simulink model "armonicosv2"  (R2017b)
settings: Solver=VariableStepAuto  StartTime=0.0  StopTime=tsim  MaxStep=stepsize  RelTol=1e-3
values from neighbouring files (symbols this model uses):
  A = blkdiag(matriz{:})    [main.m]
  C = zeros(1,n_arm*2)    [main.m]
  Fs = 500    [main.m]
  HarmonicF1 = P1(1)    [main.m]
  HarmonicF2 = P1(2)    [main.m]
  HarmonicF3 = P1(3)    [main.m]
  HarmonicF4 = P1(4)    [main.m]
  L = G    [main.m]
  n_arm = 350    [main.m]
  x0 = zeros(n_arm*2,1)    [main.m]
settings Model: Creator=choqi  LastModifiedBy=choqi

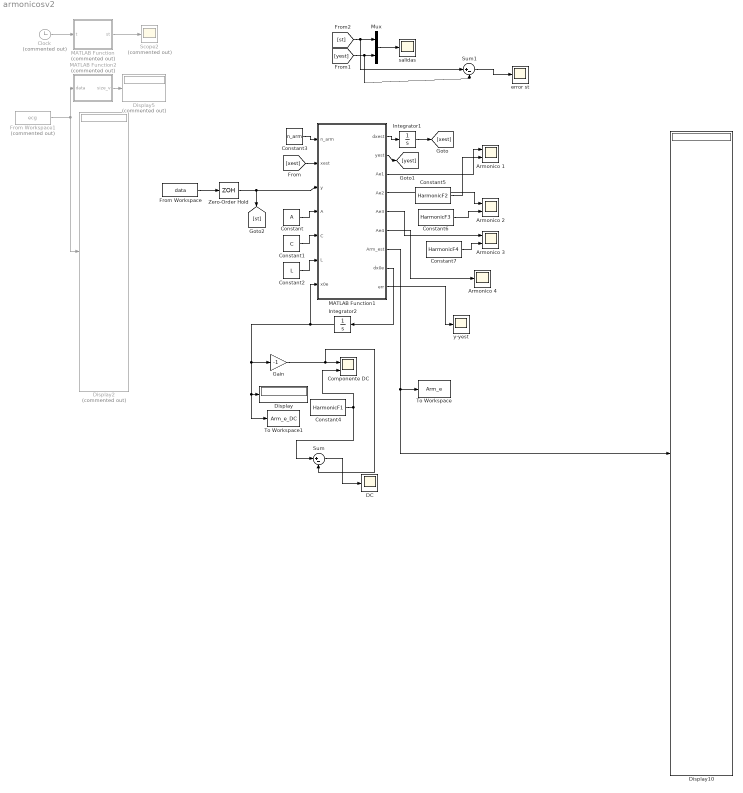
== system armonicosv2 ==
  Armonico 1 : Scope  NumInputPorts=2
  "Armonico 2 " : Scope  NumInputPorts=2
  Armonico 3 : Scope  NumInputPorts=2
  Armonico 4 : Scope
  Clock : Clock  Commented=on
  "Componente DC " : Scope  NumInputPorts=2
  Constant : Constant  Value=A
  Constant1 : Constant  Value=C
  Constant2 : Constant  Value=L
  Constant3 : Constant  Value=n_arm
  Constant4 : Constant  Value=HarmonicF1
  Constant5 : Constant  Value=HarmonicF2
  Constant6 : Constant  Value=HarmonicF3
  Constant7 : Constant  Value=HarmonicF4
  DC : Scope
  Display : Display
  Display10 : Display
  Display2 : Display  Commented=on
  Display5 : Display  Commented=on
  From Workspace : FromWorkspace  VariableName=data  SampleTime=0
  From Workspace1 : FromWorkspace  Commented=on  VariableName=ecg  SampleTime=0
  Gain : Gain  Gain=-1
  Integrator1 : Integrator  InitialCondition=x0
  Integrator2 : Integrator
  MATLAB Function : MATLAB Function  Commented=on  TreatAsAtomicUnit=on
  MATLAB Function1 : MATLAB Function  TreatAsAtomicUnit=on
  MATLAB Function2 : MATLAB Function  Commented=on  TreatAsAtomicUnit=on
  Mux : Mux  Inputs=2
  Scope2 : Scope  Commented=on
  Sum : Sum  Inputs=|+-
  Sum1 : Sum  Inputs=|+-
  To Workspace : ToWorkspace  VariableName=Arm_e  SampleTime=-1
      settings: Save2DSignal=2-D array (concatenate along first dimension)
  To Workspace1 : ToWorkspace  VariableName=Arm_e_DC  SampleTime=-1
      settings: Save2DSignal=2-D array (concatenate along first dimension)
  Zero-Order Hold : ZeroOrderHold  SampleTime=1/Fs
  error st : Scope
  salidas : Scope
  y-yest : Scope
  wires:
  MATLAB Function1/1(dxest) -> Integrator1/1
  Mux/1 -> salidas/1
  Clock/1 -> MATLAB Function/1(t)
  MATLAB Function/1(st) -> Scope2/1
  Constant2/1 -> MATLAB Function1/6(L)
  Constant/1 -> MATLAB Function1/4(A)
  Constant1/1 -> MATLAB Function1/5(C)
  [xest] -> MATLAB Function1/2(xest)
  Integrator1/1 -> [xest]
  MATLAB Function1/2(yest) -> [yest]
  From Workspace/1 -> Zero-Order Hold/1
  From Workspace1/1 -> MATLAB Function2/1(data), Display2/1
  MATLAB Function2/1(size_v) -> Display5/1
  Constant3/1 -> MATLAB Function1/1(n_arm)
  MATLAB Function1/7(Arm_est) -> Display10/1, To Workspace/1
  Zero-Order Hold/1 -> MATLAB Function1/3(y), [st]
  MATLAB Function1/3(Ae1) -> Armonico 1/1
  MATLAB Function1/4(Ae2) -> "Armonico 2 "/1
  MATLAB Function1/5(Ae3) -> Armonico 3/1
  MATLAB Function1/6(Ae4) -> Armonico 4/1
  Integrator2/1 -> Gain/1, To Workspace1/1, Display/1, MATLAB Function1/7(x0e)
  MATLAB Function1/8(dx0e) -> Integrator2/1
  Gain/1 -> Sum/2, "Componente DC "/1
  Constant4/1 -> "Componente DC "/2, Sum/1
  Constant5/1 -> Armonico 1/2
  Constant6/1 -> "Armonico 2 "/2
  Sum/1 -> DC/1
  MATLAB Function1/9(err) -> y-yest/1
  [st] -> Sum1/1, Mux/1
  Sum1/1 -> error st/1
  [yest] -> Sum1/2, Mux/2
  Constant7/1 -> Armonico 3/2

== matlab function armonicosv2/MATLAB Function1 ==
  data: n_arm input; dxest output; xest input; yest output; Ae1 output; Ae2 output; Ae3 output; Ae4 output; y input; A input; C input; L input; Arm_est output; x0e input; dx0e output; err output
function [dxest,yest,Ae1,Ae2,Ae3,Ae4,Arm_est,dx0e,err] = fcn(n_arm,xest,y,A,C,L,x0e)

yest=C'*xest+x0e;

 dx0e=38*(y-yest);
%38
 dxest=A*xest+L*(y-yest);
  Arm=zeros(1,n_arm);
err= y-yest;
for i = 1:n_arm
    j = 2*i - 1;
    Arm(i) = sqrt((C(j)^2 + C(j+1)^2)*(xest(j)^2 + xest(j+1)^2));
end
Ae1= Arm(1);
Ae2= Arm(2);
Ae3= Arm(3);
Ae4= Arm(4);
Ae5= Arm(5);
Ae6= Arm(6);
Ae7= Arm(7);
Ae8= Arm(8);
Ae9= Arm(9);
Ae10= Arm(10);
Ae11= Arm(11);
Ae12= Arm(12);
Ae13= Arm(13);
Ae14= Arm(14);
Ae15= Arm(15);
Ae16= Arm(16);
Ae17= Arm(17);
Ae18= Arm(18);
Ae19= Arm(19);
Ae20= Arm(20);
Ae21= Arm(21);
Ae22= Arm(22);
Ae23= Arm(23);
Ae24= Arm(24);
Ae25= Arm(25);
Ae26= Arm(26);
Ae27= Arm(27);
Ae28= Arm(28);
Ae29= Arm(29);
Ae30= Arm(30);
Ae31= Arm(31);
Ae32= Arm(32);
Ae33= Arm(33);
Ae34= Arm(34);
Ae35= Arm(35);
Ae36= Arm(36);
Ae37= Arm(37);
Ae38= Arm(38);
Ae39= Arm(39);
Ae40= Arm(40);
Ae41= Arm(41);
Ae42= Arm(42);
Ae43= Arm(43);
Ae44= Arm(44);
Ae45= Arm(45);
Ae46= Arm(46);
Ae47= Arm(47);
Ae48= Arm(48);
Ae49= Arm(49);
Ae50= Arm(50);
Ae51= Arm(51);
Ae52= Arm(52);
Ae53= Arm(53);
Ae54= Arm(54);
Ae55= Arm(55);
Ae56= Arm(56);
Ae57= Arm(57);
Ae58= Arm(58);
Ae59= Arm(59);
Ae60= Arm(60);
Ae61= Arm(61);
Ae62= Arm(62);
Ae63= Arm(63);
Ae64= Arm(64);
Ae65= Arm(65);
Ae66= Arm(66);
Ae67= Arm(67);
Ae68= Arm(68);


 AAA=[Ae1 Ae2 Ae3 Ae4 Ae5 Ae6 Ae7 Ae8 Ae9 Ae10...
     Ae11 Ae12 Ae13 Ae14 Ae15 Ae16 Ae17 Ae18 Ae19 Ae20...
     Ae21 Ae22 Ae23 Ae24 Ae25 Ae26 Ae27 Ae28 Ae29 Ae30...
     Ae31 Ae32 Ae33 Ae34 Ae35 Ae36 Ae37 Ae38 Ae39 Ae40...
     Ae41 Ae42 Ae43 Ae44 Ae45 Ae46 Ae47 Ae48 Ae49 Ae50...
     Ae51 Ae52 Ae53 Ae54 Ae55 Ae56 Ae57 Ae58 Ae59 Ae60...
     Ae61 Ae62 Ae63 Ae64 Ae65 Ae66 Ae67 Ae68 ];
%AAA=[Ae1 Ae2 Ae3];
Arm_est=AAA';
%  Ae1 = sqrt((C(1)^2 + C(2)^2)*(xest(1)^2 + xest(2)^2));
%  Ae2 = sqrt((C(3)^2 + C(4)^2)*(xest(3)^2 + xest(4)^2));
 % Ae3 = sqrt((C(5)^2 + C(6)^2)*(xest(5)^2 + xest(6)^2));
  %Ae4 = sqrt((C(7)^2 + C(8)^2)*(xest(7)^2 + xest(8)^2));
% Ae5 = sqrt((k9^2 + k10^2)*(xest(9)^2 + xest(10)^2));
% Ae6 = sqrt((k11^2 + k12^2)*(xest(11)^2 + xest(12)^2));
% Ae7 = sqrt((k13^2 + k14^2)*(xest(13)^2 + xest(14)^2));
% Ae8 = sqrt((k15^2 + k16^2)*(xest(15)^2 + xest(16)^2));
% Ae9 = sqrt((k17^2 + k18^2)*(xest(17)^2 + xest(18)^2));
% Ae10 = sqrt((k19^2 + k20^2)*(xest(19)^2 + xest(20)^2));
% Ae11 = sqrt((k21^2 + k22^2)*(xest(21)^2 + xest(22)^2));
% Ae12 = sqrt((k23^2 + k24^2)*(xest(23)^2 + xest(24)^2));
% Ae13 = sqrt((k25^2 + k26^2)*(xest(25)^2 + xest(26)^2));
% Ae14 = sqrt((k27^2 + k28^2)*(xest(27)^2 + xest(28)^2));
% Ae15 = sqrt((k29^2 + k30^2)*(xest(29)^2 + xest(30)^2));
% Ae16 = sqrt((k31^2 + k32^2)*(xest(31)^2 + xest(32)^2));
% Ae17 = sqrt((k33^2 + k34^2)*(xest(33)^2 + xest(34)^2));
% Ae18 = sqrt((k35^2 + k36^2)*(xest(35)^2 + xest(36)^2));
% Ae19 = sqrt((k37^2 + k38^2)*(xest(37)^2 + xest(38)^2));
% Ae20 = sqrt((k39^2 + k40^2)*(xest(39)^2 + xest(40)^2));
% Ae21 = sqrt((k41^2 + k42^2)*(xest(41)^2 + xest(42)^2));
% Ae22 = sqrt((k43^2 + k44^2)*(xest(43)^2 + xest(44)^2));
% Ae23 = sqrt((k45^2 + k46^2)*(xest(45)^2 + xest(46)^2));
% Ae24 = sqrt((k47^2 + k48^2)*(xest(47)^2 + xest(48)^2));
% Ae25 = sqrt((k49^2 + k50^2)*(xest(49)^2 + xest(50)^2));
% Ae26 = sqrt((k51^2 + k52^2)*(xest(51)^2 + xest(52)^2));
% Ae27 = sqrt((k53^2 + k54^2)*(xest(53)^2 + xest(54)^2));
% Ae28 = sqrt((k55^2 + k56^2)*(xest(55)^2 + xest(56)^2));
% Ae29 = sqrt((k57^2 + k58^2)*(xest(57)^2 + xest(58)^2));
% Ae30 = sqrt((k59^2 + k60^2)*(xest(59)^2 + xest(60)^2));
% Ae31 = sqrt((k61^2 + k62^2)*(xest(61)^2 + xest(62)^2));
% Ae32 = sqrt((k63^2 + k64^2)*(xest(63)^2 + xest(64)^2));
% Ae33 = sqrt((k65^2 + k66^2)*(xest(65)^2 + xest(66)^2));
% Ae34 = sqrt((k67^2 + k68^2)*(xest(67)^2 + xest(68)^2));
% Ae35 = sqrt((k69^2 + k70^2)*(xest(69)^2 + xest(70)^2));
% Ae36 = sqrt((k71^2 + k72^2)*(xest(71)^2 + xest(72)^2));
% Ae37 = sqrt((k73^2 + k74^2)*(xest(73)^2 + xest(74)^2));
% Ae38 = sqrt((k75^2 + k76^2)*(xest(75)^2 + xest(76)^2));
% Ae39 = sqrt((k77^2 + k78^2)*(xest(77)^2 + xest(78)^2));
% Ae40 = sqrt((k79^2 + k80^2)*(xest(79)^2 + xest(80)^2));
% Ae41 = sqrt((k81^2 + k82^2)*(xest(81)^2 + xest(82)^2));
% Ae42 = sqrt((k83^2 + k84^2)*(xest(83)^2 + xest(84)^2));
% Ae43 = sqrt((k85^2 + k86^2)*(xest(85)^2 + xest(86)^2));
% Ae44 = sqrt((k87^2 + k88^2)*(xest(87)^2 + xest(88)^2));
% Ae45 = sqrt((k89^2 + k90^2)*(xest(89)^2 + xest(90)^2));
% Ae46 = sqrt((k91^2 + k92^2)*(xest(91)^2 + xest(92)^2));
% Ae47 = sqrt((k93^2 + k94^2)*(xest(93)^2 + xest(94)^2));
% Ae48 = sqrt((k95^2 + k96^2)*(xest(95)^2 + xest(96)^2));
% Ae49 = sqrt((k97^2 + k98^2)*(xest(97)^2 + xest(98)^2));
% Ae50 = sqrt((k99^2 + k100^2)*(xest(99)^2 + xest(100)^2));
% Ae51 = sqrt((k101^2 + k102^2)*(xest(101)^2 + xest(102)^2));
% Ae52 = sqrt((k103^2 + k104^2)*(xest(103)^2 + xest(104)^2));
% Ae53 = sqrt((k105^2 + k106^2)*(xest(105)^2 + xest(106)^2));
% Ae54 = sqrt((k107^2 + k108^2)*(xest(107)^2 + xest(108)^2));
% Ae55 = sqrt((k109^2 + k110^2)*(xest(109)^2 + xest(110)^2));
% Ae56 = sqrt((k111^2 + k112^2)*(xest(111)^2 + xest(112)^2));
% Ae57 = sqrt((k113^2 + k114^2)*(xest(113)^2 + xest(114)^2));
% Ae58 = sqrt((k115^2 + k116^2)*(xest(115)^2 + xest(116)^2));
% Ae59 = sqrt((k117^2 + k118^2)*(xest(117)^2 + xest(118)^2));
% Ae60 = sqrt((k119^2 + k120^2)*(xest(119)^2 + xest(120)^2));
% Ae61 = sqrt((k121^2 + k122^2)*(xest(121)^2 + xest(122)^2));
% Ae62 = sqrt((k123^2 + k124^2)*(xest(123)^2 + xest(124)^2));
% Ae63 = sqrt((k125^2 + k126^2)*(xest(125)^2 + xest(126)^2));
% Ae64 = sqrt((k127^2 + k128^2)*(xest(127)^2 + xest(128)^2));
% Ae65 = sqrt((k129^2 + k130^2)*(xest(129)^2 + xest(130)^2));
% Ae66 = sqrt((k131^2 + k132^2)*(xest(131)^2 + xest(132)^2));
% Ae67 = sqrt((k133^2 + k134^2)*(xest(133)^2 + xest(134)^2));
% Ae68 = sqrt((k135^2 + k136^2)*(xest(135)^2 + xest(136)^2));

== matlab function armonicosv2/MATLAB Function ==
  data: st output; t input
function st  = fcn(t)

w=0.9;
A1 = 0.5;
A2 = 0.1;
A3 = 0.9;
A4 = 0.2;
A5 = 0.05;
A6 = 0.3;
A7 = 0.7;
A8 = 0.95;
theta1 = 0;
theta2 = 0;
%st = A1*sin(w*t + theta1) + A2*sin(2*w*t + theta2) + A3*sin(3*w*t) + A4*sin(4*w*t)+...
   %  A5*sin(5*w*t) + A6*sin(6*w*t)+ A7*sin(7*w*t) + A8*sin(8*w*t);

 %st = A1*sin(w*t + theta1) + A2*sin(2*w*t + theta2) + A3*sin(3*w*t)+ A4*sin(4*w*t);
 st = 1.2*sin(2*pi*1.7*t) + 0.5*sin(2*pi*1.2*t) + 0.3*sin(2*pi*3.1*t);
%st = st1 + 0.05*randn(size(t));

== matlab function armonicosv2/MATLAB Function2 ==
  data: size_v output; data input
function size_v = a(data)
    size_v = size(data);
end
